simulink library "INT_RailP_VDGradMon"  (R2016b)
settings: Solver=VariableStepAuto  StartTime=0.0  StopTime=10.0  RelTol=1e-3
settings Model: Creator=Administrator  LastModifiedBy=Administrator

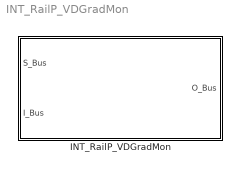
== system INT_RailP_VDGradMon ==
  INT_RailP_VDGradMon : Subsystem

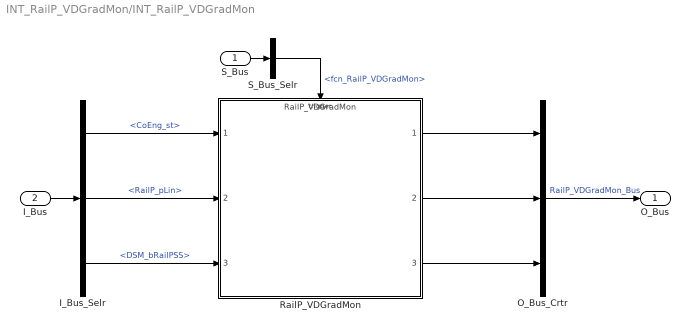
== system INT_RailP_VDGradMon/INT_RailP_VDGradMon ==
  S_Bus : Inport
  I_Bus : Inport  Port=2
  I_Bus_Selr : BusSelector  OutputSignals=CoEng_st,RailP_pLin,DSM_bRailPSS
  O_Bus_Crtr : BusCreator  Inputs=3
  RailP_VDGradMon : ModelReference  ModelNameDialog=RailP_VDGradMon  SimulationMode=Normal  ModelReferenceVersion=1.18  TriggerPortName=function  TriggerPortTriggerType=function-call  TriggerPortStatesWhenEnabling=held
  S_Bus_Selr : BusSelector  OutputSignals=fcn_RailP_VDGradMon
  O_Bus : Outport
  wires:
  S_Bus_Selr/1 -> RailP_VDGradMon/Trigger  "<fcn_RailP_VDGradMon>"
  S_Bus/1 -> S_Bus_Selr/1
  I_Bus/1 -> I_Bus_Selr/1
  I_Bus_Selr/1 -> RailP_VDGradMon/1  "<CoEng_st>"
  I_Bus_Selr/2 -> RailP_VDGradMon/2  "<RailP_pLin>"
  I_Bus_Selr/3 -> RailP_VDGradMon/3  "<DSM_bRailPSS>"
  O_Bus_Crtr/1 -> O_Bus/1  "RailP_VDGradMon_Bus"
  RailP_VDGradMon/1 -> O_Bus_Crtr/1
  RailP_VDGradMon/2 -> O_Bus_Crtr/2
  RailP_VDGradMon/3 -> O_Bus_Crtr/3
